simulink model "sgMdl_IO144_AnalogDigitalLoopback"  (R2024b)
settings: Solver=FixedStepAuto  StartTime=0.0  StopTime=inf  RelTol=1e-3  EnableMultiTasking=on
libraries: speedgoatlib_IO144 x4
Description:
  | IO144 - Analog Output and Digital Loopback
settings Model: ModifiedByFormat=Speedgoat  SimulationMode=external  ExtModeEnableFloating=off  ExtModeTrigDuration=100000  Creator=Speedgoat  LastModifiedBy=Speedgoat
settings SolverCC: ConcurrentTasks=on  AlgebraicLoopSolver=TrustRegion  PositivePriorityOrder=on
settings DataIOCC: SaveFormat=StructureWithTime  ReturnWorkspaceOutputs=off
settings OptimizationCC: BlockReduction=off  OptimizeBlockIOStorage=off  BufferReuse=off  ReuseModelBlockBuffer=off  GlobalBufferReuse=off  ExpressionFolding=off  LocalBlockOutputs=off
settings DebuggingCC: TasksWithSamePriorityMsg=none  UnconnectedInputMsg=warning  UnconnectedOutputMsg=warning  UnconnectedLineMsg=warning  SFExecutionAtInitializationDiag=none  ArithmeticOperatorsInVariantConditions=warning
settings HardwareCC: ProdBitPerLong=64  ProdLongLongMode=on  ProdHWDeviceType=Intel->x86-64 (Linux 64)
settings ModelReferenceCC: EnableRefExpFcnMdlSchedulingChecks=on
settings SFSimCC: SimUseLocalCustomCode=off  CustomCodeUndefinedFunction=UseInterfaceOnly
settings RTWCC: Description=Speedgoat Real-Time Target Machine  SystemTargetFile=speedgoat.tlc  TemplateMakefile=slrealtime_default_tmf  RTWUseLocalCustomCode=off  Toolchain=Simulink Real-Time Toolchain  BuildConfiguration=Faster Runs  TargetLang=C++  GPUComputeCapability=3.5  DLArmComputeVersion=19.05
settings CodeAppCC: StateflowObjectComments=on
settings SimulinkRealTimeTargetCC: SubcomponentCodeInterfacePackaging=Reusable function  InstructionSetFMA=off  LogToMDFFile=off  SLRTFileLogMaxRuns=10  UseGCCFastMath=on
settings ConfigComp: CovBoundaryAbsTol=1.0e-5
settings SimscapeCC: SimscapeNormalizeSystem=off

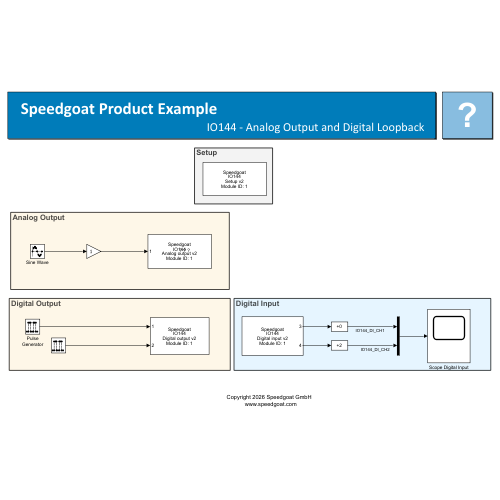
[thumbnail: Simulink's stored preview of the top-level diagram]
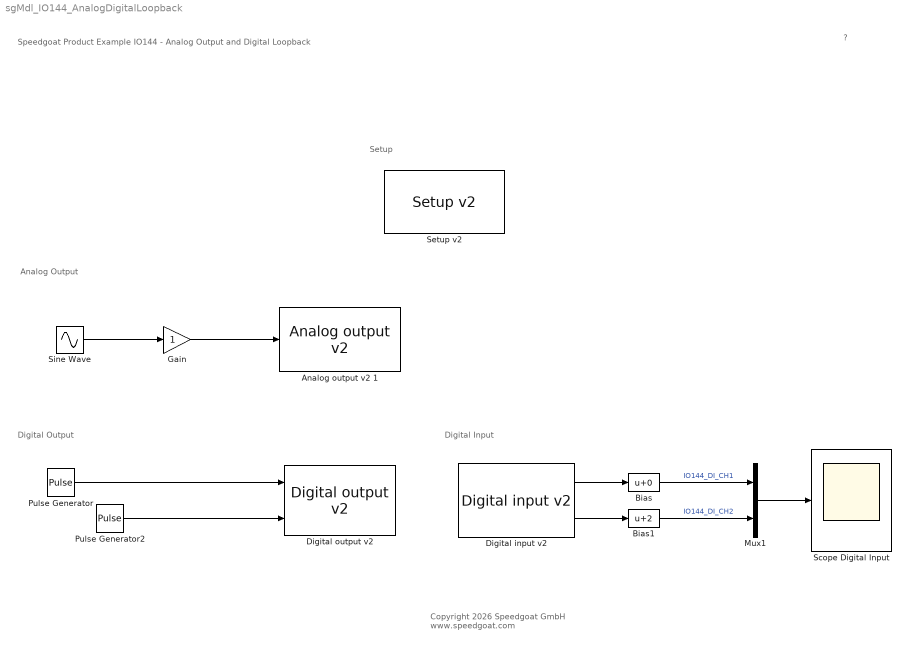
== system sgMdl_IO144_AnalogDigitalLoopback ==
  note: Digital Input
  note: Digital Output
  note: Setup
  note: Analog Output
  note: Speedgoat Product Example
      | IO144 - Analog Output and Digital Loopback
  note: ?
  note: Copyright 2026 Speedgoat GmbH
      |  www.speedgoat.com
  Analog output v2 1 : speedgoatlib_IO144/Analog output v2   parModuleId=1  parTs=-1  parPciSlot=-1  parUseDMA=off  parDaSyncOut=on  parDaChannels=1  parDaInitValue=0  parDaReset=1  parDaFrameSize=1  parDaRange=[4 0 0 0 0 0 0 0 0 0 0 0 0 0 0 0]
      settings: SourceProductName=Simulink Real-Time: Speedgoat I/O Blockset
  Bias : Bias  SaturateOnIntegerOverflow=off
  Bias1 : Bias  Bias=2  SaturateOnIntegerOverflow=off
  "Digital input v2 " : speedgoatlib_IO144/Digital input v2   parModuleId=1  parTs=-1  parPciSlot=-1  parDiChannels=[3 4]
      settings: SourceProductName=Simulink Real-Time: Speedgoat I/O Blockset
  "Digital output v2 " : speedgoatlib_IO144/Digital output v2   parModuleId=1  parTs=-1  parDoChannels=[1 2]  parDoInitValues=[0 0]  parDoReset=[1 1]  parPciSlot=-1  parIOPullReferenceFront=Pull-up 3.3 V  parIOPullReferenceRear=Floating
      settings: SourceProductName=Simulink Real-Time: Speedgoat I/O Blockset
  Gain : Gain
  Mux1 : Mux  Inputs=2
  Pulse Generator : DiscretePulseGenerator  Period=25  PulseWidth=5  SampleTime=0.001
  Pulse Generator2 : DiscretePulseGenerator  Period=25  PulseWidth=10  SampleTime=0.001
  Scope Digital Input : Scope
  "Setup v2 " : speedgoatlib_IO144/Setup v2   parPciSlot=-1  parModuleId=1  parCalibrate=on  parUseDMA=off  parDaSyncOut=on  parDaChannels=[1]  parDaInitValue=0  parDaReset=1  parDaRange1=+-10 V  parDaRange2=0-5 V  parDaRange3=0-5 V  parDaRange4=0-5 V  parDaRange5=0-5 V  parDaRange6=0-5 V  parDaRange7=0-5 V  parDaRange8=0-5 V  parDaRange9=0-5 V  parDaRange10=0-5 V  parDaRange11=0-5 V  parDaRange12=0-5 V  parDaRange13=0-5 V  parDaRange14=0-5 V  parDaRange15=0-5 V  parDaRange16=0-5 V  parDaRange=[4 0 0 0 0 0 0 0 0 0 0 0 0 0 0 0]  parDaClockSource=Self Clocked  parDaClockRate=20MHz  parDaClockDivider=20000  parDaSampleTime=1.000000000e-03  parDaEnClkOutput=Disabled  parDaFrameSize=1  parDaTriggerSource=Self Clocked  parDaTriggerMultiplier=10  parDaTriggerTime=5.000000000e-07  parDaEnTriggerOutput=Disabled  parDoChannels=[1 2]  parDoInitValues=0  parDoReset=1  parDiChannels=[3 4]  parIOPullReferenceFront=Pull-up 3.3 V  parIOPullReferenceRear=Floating
      settings: SourceProductName=Simulink Real-Time: Speedgoat I/O Blockset
  Sine Wave : Sin  SineType=Sample based  Amplitude=2  Frequency=2*pi*5  Samples=50  SampleTime=0.001
  wires:
  Gain/1 -> Analog output v2 1/1
  Sine Wave/1 -> Gain/1
  Pulse Generator2/1 -> "Digital output v2 "/2
  Pulse Generator/1 -> "Digital output v2 "/1
  Mux1/1 -> Scope Digital Input/1
  Bias/1 -> Mux1/1  "IO144_DI_CH1"
  Bias1/1 -> Mux1/2  "IO144_DI_CH2"
  "Digital input v2 "/1 -> Bias/1
  "Digital input v2 "/2 -> Bias1/1
